simulink model "RC_circuit"  (R2021a)
settings: Solver=VariableStepAuto  StartTime=0.0  StopTime=10.0  MaxStep=1e-3  RelTol=1e-3
settings Model: Creator=YasserNet  LastModifiedBy=YasserNet

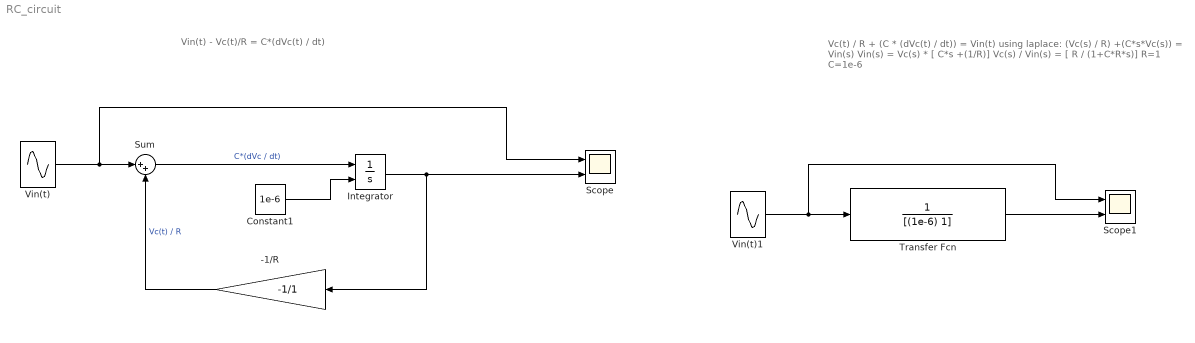
== system RC_circuit ==
  note: Vc(t) / R + (C * (dVc(t) / dt)) = Vin(t)
      | using laplace: (Vc(s) / R) +(C*s*Vc(s)) = Vin(s)
      | Vin(s) = Vc(s) * [ C*s +(1/R)]
      | Vc(s) / Vin(s) = [ R / (1+C*R*s)]
      | R=1
      | C=1e-6
  note: Vin(t) - Vc(t)/R = C*(dVc(t) / dt)
  -1/R : Gain  Gain=-1/1
  Constant1 : Constant  Value=1e-6
  Integrator : Integrator  InitialConditionSource=external  InitialCondition=1
  Scope : Scope  NumInputPorts=2
  Scope1 : Scope  NumInputPorts=2
  Sum : Sum  Inputs=|++
  Transfer Fcn : TransferFcn  Denominator=[(1e-6) 1]
  Vin(t) : Sin  Amplitude=5  Frequency=2*pi  SampleTime=0
  Vin(t)1 : Sin  Amplitude=5  Frequency=2*pi  SampleTime=0
  wires:
  Vin(t)/1 -> Scope/1, Sum/1
  -1/R/1 -> Sum/2  "Vc(t) / R"
  Sum/1 -> Integrator/1  "C*(dVc / dt)"
  Integrator/1 -> -1/R/1, Scope/2
  Constant1/1 -> Integrator/2
  Vin(t)1/1 -> Scope1/1, Transfer Fcn/1
  Transfer Fcn/1 -> Scope1/2
